simulink model "mission_manager"  (R2023b)
settings: Solver=VariableStepAuto  StartTime=0.0  StopTime=inf  RelTol=1e-3
undefined symbols (not defined in the file or in its folder): depth, x_cmd, y_cmd, yaw
libraries: ros2lib x3
settings Model: Creator=donjoe  LastModifiedBy=donjoe

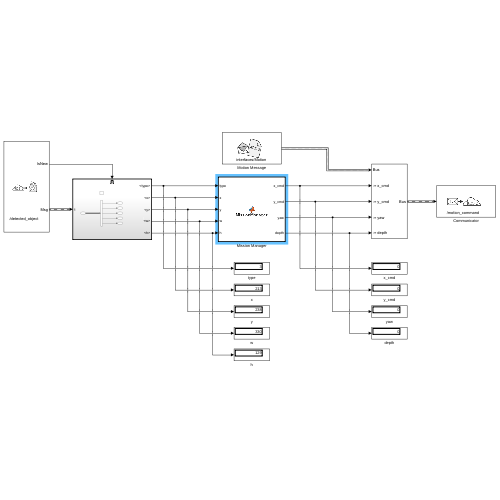
[thumbnail: Simulink's stored preview of the top-level diagram]
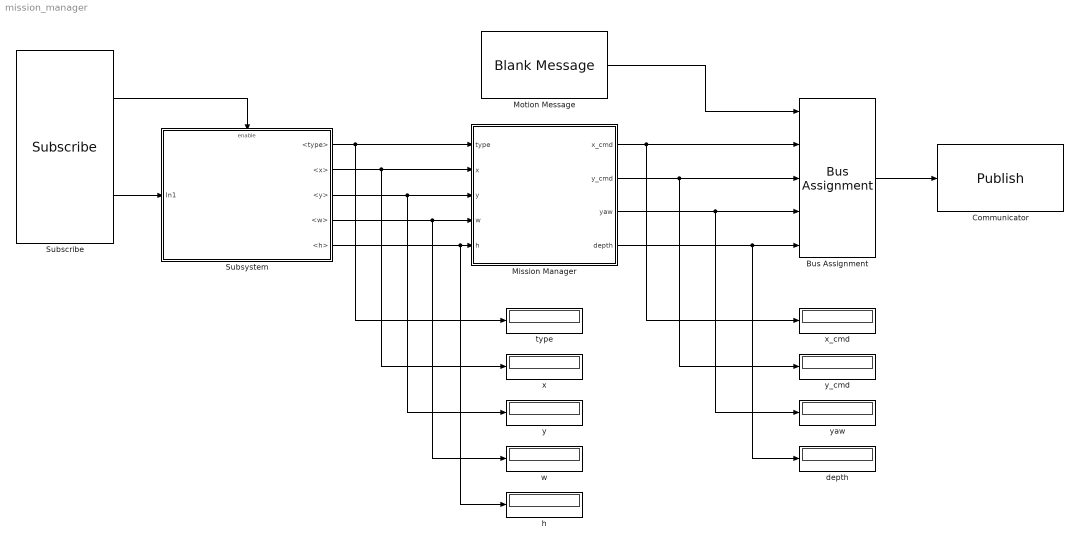
== system mission_manager ==
  Bus Assignment : BusAssignment  AssignedSignals=x_cmd,y_cmd,yaw,depth
  Communicator : ros2lib/Publish  topicSource=Specify your own  topic=/motion_command  messageType=interfaces/Motion  QOSHistory=Keep last  QOSDepth=1  QOSReliability=Reliable  QOSDurability=Volatile
  Mission Manager : MATLAB Function  TreatAsAtomicUnit=on
  Motion Message : ros2lib/Blank Message  messageClass=Message  entityType=interfaces/Motion  messageType=interfaces/Motion  SampleTime=1
  Subscribe : ros2lib/Subscribe  topicSource=Specify your own  topic=/detected_object  messageType=interfaces/Object  sampleTime=1  QOSHistory=Keep last  QOSDepth=1  QOSReliability=Reliable  QOSDurability=Volatile
  Subsystem : Subsystem
  depth : Display
  h : Display
  type : Display
  w : Display
  x : Display
  x_cmd : Display
  y : Display
  y_cmd : Display
  yaw : Display
  wires:
  Bus Assignment/1 -> Communicator/1
  Motion Message/1 -> Bus Assignment/1
  Mission Manager/1(x_cmd) -> Bus Assignment/2, x_cmd/1
  Mission Manager/2(y_cmd) -> Bus Assignment/3, y_cmd/1
  Mission Manager/3(yaw) -> Bus Assignment/4, yaw/1
  Mission Manager/4(depth) -> Bus Assignment/5, depth/1
  Subscribe/2 -> Subsystem/1(In1)
  Subsystem/1(<type>) -> Mission Manager/1(type), type/1
  Subsystem/2(<x>) -> Mission Manager/2(x), x/1
  Subscribe/1 -> Subsystem/Enable
  Subsystem/3(<y>) -> Mission Manager/3(y), y/1
  Subsystem/4(<w>) -> Mission Manager/4(w), w/1
  Subsystem/5(<h>) -> h/1, Mission Manager/5(h)

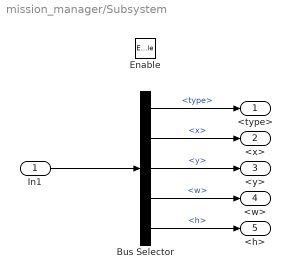
== system mission_manager/Subsystem ==
  In1 : Inport
  Enable : EnablePort
  Bus Selector : BusSelector  OutputSignals=type,x,y,w,h
  <type> : Outport
  <x> : Outport  Port=2
  <y> : Outport  Port=3
  <w> : Outport  Port=4
  <h> : Outport  Port=5
  wires:
  Bus Selector/3 -> <y>/1  "<y>"
  In1/1 -> Bus Selector/1
  Bus Selector/2 -> <x>/1  "<x>"
  Bus Selector/1 -> <type>/1  "<type>"
  Bus Selector/4 -> <w>/1  "<w>"
  Bus Selector/5 -> <h>/1  "<h>"

== matlab function mission_manager/Mission Manager ==
  data: type input; x_cmd output; x input; y input; y_cmd output; yaw output; depth output; w input; h input
function [x_cmd, y_cmd, yaw, depth] = MissionManager(type, x, y, w, h)

persistent target;
if isempty(target)
    target = 1;
end

x_cmd = int32(0);
y_cmd = int32(0);
yaw = int32(0);
depth = int32(0);

disp(target)

if type == 0 || target == type
    % fprintf("Moving to target %d", int32(type));
    % printf("Moving to target %d", int32(type));
    x_cmd = x;
    depth = y;
    if -10 < x_cmd && x_cmd < 10 && -10 < y_cmd && y_cmd < 10
        y_cmd = int32(500);
    end
    if type ~= 0 && w > 640 && h > 640       
        target = target + 1;
    end
elseif target > 3
    disp("Done")
else
    disp("gada apapa")
    % printf("Non-target found '%d', skipping\n", int32(type));
end
